simulink model "Verifikation_Dyn_R2019b"  (R2023a)
settings: Solver=ode5  StartTime=0.0  StopTime=10.0  FixedStep=Ta  RelTol=1e-3
values from neighbouring files (symbols this model uses):
  params_CRS = [g m2 m3 s2 s3 l2 l3 B_S1 A_S2 B_S2 C_S2 A_S3 B_S3 C_S3 i_G1 i_G2 i_G3 B_M1 C_M2 C_M3]    [init_CRS255_ss.m]
  x1_ic = zeros(6,1)    [init_CRS255_ss.m]
settings Model: Creator=Hoebarth  LastModifiedBy=Flo
settings SolverCC: AlgebraicLoopSolver=TrustRegion
settings DataIOCC: LimitDataPoints=on  SaveFormat=Array  SignalLoggingSaveFormat=ModelDataLogs  ReturnWorkspaceOutputs=off  SignalLoggingName=sigsOut
settings OptimizationCC: BooleanDataType=off  OptimizeBlockIOStorage=off  BufferReuse=off  GlobalBufferReuse=off  ExpressionFolding=off  ExpressionDepthLimit=2147483647  LocalBlockOutputs=off  InitFltsAndDblsToZero=on  LifeSpan=inf  OptimizeDataStoreBuffers=off  BusAssignmentInplaceUpdate=off
settings DebuggingCC: SaveWithParameterizedLinksMsg=none  UnderspecifiedInitializationDetection=Classic  MergeDetectMultiDrivingBlocksExec=none  SignalResolutionControl=TryResolveAllWithWarning  MultiTaskDSMMsg=warning  MultiTaskCondExecSysMsg=none  FcnCallInpInsideContextMsg=warning  UnconnectedInputMsg=warning  UnconnectedOutputMsg=warning  UnconnectedLineMsg=warning  StateNameClashWarn=warning  SFUnexpectedBacktrackingDiag=warning  SFNoUnconditionalDefaultTransitionDiag=warning  SFExecutionAtInitializationDiag=none  ArithmeticOperatorsInVariantConditions=warning
settings HardwareCC: ProdBitPerPointer=32  ProdBitPerSizeT=32  ProdBitPerPtrDiffT=32  ProdLargestAtomicFloat=None  ProdIntDivRoundTo=Undefined  ProdEndianess=Unspecified  ProdWordSize=32  ProdHWDeviceType=32-bit Generic  TargetUnknown=on
settings ModelReferenceCC: EnableRefExpFcnMdlSchedulingChecks=on  PropagateSignalLabelsOutOfModel=off
settings SFSimCC: SimUseLocalCustomCode=off  CustomCodeUndefinedFunction=UseInterfaceOnly
settings RTWCC: MakeCommand=make_wc  GenerateMakefile=off  TemplateMakefile=nt_msvc.tmf  RTWUseLocalCustomCode=off
settings CodeAppCC: StateflowObjectComments=on
settings GRTTargetCC: TargetFcnLib=ansi_tfl_tmw.mat  TargetLangStandard=C89/C90 (ANSI)  ModelReferenceCompliant=off  CompOptLevelCompliant=off  CombineOutputUpdateFcns=off  MatFileLogging=off  GRTInterface=on  UseToolchainInfoCompliant=off
settings ConfigComp: CovMetricSettings=dw  CovSaveCumulativeToWorkspaceVar=on  CovSaveSingleToWorkspaceVar=on  CovExternalEMLEnable=off

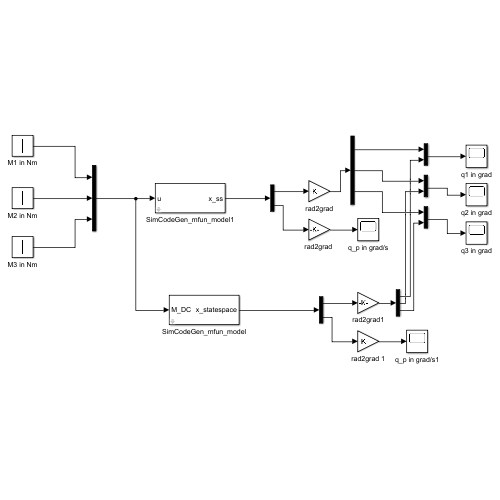
[thumbnail: Simulink's stored preview of the top-level diagram]
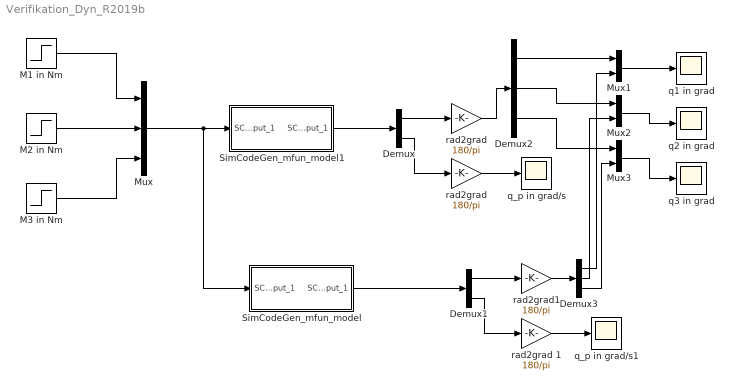
== system Verifikation_Dyn_R2019b ==
  Demux : Demux  Outputs=[3,3]
  Demux1 : Demux  Outputs=[3,3]
  Demux2 : Demux  Outputs=3
  Demux3 : Demux  Outputs=3
  M1 in Nm : Step  Before=0.001  After=0  SampleTime=0
  M2 in Nm : Step  Time=2  Before=0.001  After=0  SampleTime=0
  M3 in Nm : Step  Time=3  Before=0.001  After=0  SampleTime=0
  Mux : Mux  Inputs=3
  Mux1 : Mux  Inputs=2
  Mux2 : Mux  Inputs=2
  Mux3 : Mux  Inputs=2
  SimCodeGen_mfun_model : Subsystem  mask{SC_param_0=params_CRS, SC_x1_ic=x1_ic}
      mask prompts: SC_param_0 "params_CRS"
      mask Display:
      | port_label('input', 1, 'M_DC');
      | port_label('output', 1, 'x_statespace');
  SimCodeGen_mfun_model1 : Subsystem  mask{SC_param_0=params_CRS, SC_x1_ic=x1_ic}
      mask prompts: SC_param_0 "params_CRS"
      mask Display:
      | port_label('input', 1, 'u');
      | port_label('output', 1, 'x_ss');
  q1 in grad : Scope
  q2 in grad : Scope
  q3 in grad : Scope
  q_p in grad/s : Scope
  q_p in grad/s1 : Scope
  rad2grad : Gain  Gain=180/pi
  "rad2grad " : Gain  Gain=180/pi
  rad2grad 1 : Gain  Gain=180/pi
  rad2grad1 : Gain  Gain=180/pi
  wires:
  M1 in Nm/1 -> Mux/1
  M2 in Nm/1 -> Mux/2
  M3 in Nm/1 -> Mux/3
  Mux/1 -> SimCodeGen_mfun_model1/1(SC_input_1), SimCodeGen_mfun_model/1(SC_input_1)
  SimCodeGen_mfun_model1/1(SC_output_1) -> Demux/1
  Demux/1 -> rad2grad/1
  Demux/2 -> "rad2grad "/1
  "rad2grad "/1 -> q_p in grad/s/1
  rad2grad 1/1 -> q_p in grad/s1/1
  Demux1/2 -> rad2grad 1/1
  Demux1/1 -> rad2grad1/1
  SimCodeGen_mfun_model/1(SC_output_1) -> Demux1/1
  rad2grad/1 -> Demux2/1
  Demux2/1 -> Mux1/1
  Demux3/1 -> Mux1/2
  rad2grad1/1 -> Demux3/1
  Mux1/1 -> q1 in grad/1
  Demux2/2 -> Mux2/1
  Demux2/3 -> Mux3/1
  Demux3/2 -> Mux2/2
  Demux3/3 -> Mux3/2
  Mux2/1 -> q2 in grad/1
  Mux3/1 -> q3 in grad/1

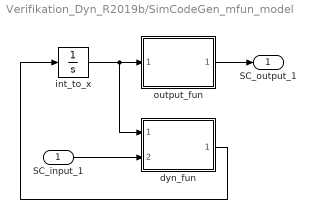
== system Verifikation_Dyn_R2019b/SimCodeGen_mfun_model ==
  SC_input_1 : Inport
  dyn_fun : MATLAB Function  TreatAsAtomicUnit=on
  int_to_x : Integrator  InitialCondition=[SC_x1_ic]
  output_fun : MATLAB Function  TreatAsAtomicUnit=on
  SC_output_1 : Outport
  wires:
  dyn_fun/1(SC_state_dot) -> int_to_x/1
  output_fun/1(SC_output_0) -> SC_output_1/1
  SC_input_1/1 -> dyn_fun/2(SC_input_0)
  int_to_x/1 -> output_fun/1(SC_state), dyn_fun/1(SC_state)

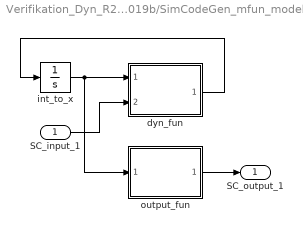
== system Verifikation_Dyn_R2019b/SimCodeGen_mfun_model1 ==
  SC_input_1 : Inport
  dyn_fun : MATLAB Function  TreatAsAtomicUnit=on
  int_to_x : Integrator  InitialCondition=[SC_x1_ic]
  output_fun : MATLAB Function  TreatAsAtomicUnit=on
  SC_output_1 : Outport
  wires:
  output_fun/1(SC_output_0) -> SC_output_1/1
  int_to_x/1 -> output_fun/1(SC_state), dyn_fun/1(SC_state)
  SC_input_1/1 -> dyn_fun/2(SC_input_0)
  dyn_fun/1(SC_state_dot) -> int_to_x/1

== matlab function Verifikation_Dyn_R2019b/SimCodeGen_mfun_model/dyn_fun ==
  data: SC_state input size=[6]; SC_state_dot output size=[6]; SC_input_0 input size=[3]; SC_param_0 parameter
function SC_state_dot  = dyn_fun(SC_state, SC_input_0, SC_param_0)
    SC_state_dot = zeros(6, 1);
    SC_state_x_0 = SC_state(1:6);
    SC_eval = zeros(6,1);
    SC_eval(1) = SC_state_x_0(4);
    SC_eval(2) = SC_state_x_0(5);
    SC_eval(3) = SC_state_x_0(6);
    t1 = SC_state_x_0(2);
    t2 = cos(t1);
    t3 = t2 ^ 2;
    t4 = SC_param_0(6);
    t5 = t4 ^ 2;
    t7 = SC_param_0(3);
    t9 = SC_param_0(2);
    t11 = SC_param_0(4);
    t12 = t11 ^ 2;
    t14 = sin(t1);
    t15 = SC_state_x_0(3);
    t16 = cos(t15);
    t19 = SC_param_0(5);
    t23 = t16 ^ 2;
    t25 = t19 ^ 2;
    t27 = SC_param_0(9);
    t29 = SC_param_0(12);
    t31 = SC_param_0(15);
    t32 = t31 ^ 2;
    t35 = SC_param_0(10);
    t37 = SC_param_0(13);
    t39 = t7 * t5;
    t40 = t9 * t12;
    t18 = t9 * t12;
    t21 = t25 * t7;
    t24 = t7 * t5;
    t42 = 0.2e1 * t14 * t16 * t19 * t4 * t7 - t18 * t3 + t21 * t23 - t23 * t29 + t23 * t37 - t24 * t3 + t27 * t3 - t3 * t35 + t32 * SC_param_0(18) + t29 + t35 + t39 + t40 + SC_param_0(8);
    t43 = SC_eval(2);
    t46 = t43 * t2;
    t50 = t27 * t43;
    t44 = SC_eval(1);
    t51 = t14 * t44;
    t53 = t43 * t35;
    t55 = SC_param_0(11);
    t56 = t55 * t43;
    t60 = t2 * t44;
    t68 = t14 * t4 + t16 * t19;
    t71 = sin(t15);
    t76 = t16 * t44;
    t78 = t1 + t15;
    t79 = cos(t78);
    t80 = t4 * t79;
    t81 = t80 * t43;
    t83 = t71 * t44;
    t84 = sin(t78);
    t85 = t4 * t84;
    t86 = t85 * t43;
    t48 = SC_eval(3);
    t88 = t19 * t48 - t86;
    t93 = t29 * t48;
    t95 = t48 * t37;
    t97 = SC_param_0(14);
    t98 = t97 * t48;
    SC_eval(4) = 0.1e1 / t42 * (-0.2e1 * t14 * t18 * t46 * t44 + (t50 * t51 - t51 * t53 + t51 * t56) * t2 + (t50 * t60 - t53 * t60 - t56 * t60) * t14 - t68 * (t7 * t44 * (-t19 * t48 * t71 + t4 * t46) + t81 * t7 * t76 - t88 * t7 * t83) + (-t76 * t93 + t76 * t95 - t76 * t98) * t71 + (-t83 * t93 + t83 * t95 + t83 * t98) * t16 + SC_input_0(1) * t31);
    t110 = t25 * t7;
    t111 = SC_param_0(17);
    t112 = t111 ^ 2;
    t113 = SC_param_0(20);
    t114 = t113 * t112;
    t116 = t84 ^ 2;
    t118 = t7 ^ 2;
    t121 = SC_param_0(19);
    t123 = SC_param_0(16);
    t124 = t123 ^ 2;
    t127 = t121 * t124;
    t125 = t25 * t118;
    t147 = t112 * t113 * t121 * t124 + t12 * t25 * t7 * t9 + t112 * t113 * t55 - t116 * t125 * t5 + t121 * t124 * t97 + t110 * t127 + t114 * t39 + t114 * t40 + t125 * t5 + t18 * t97 + t21 * t55 + t24 * t97 + t55 * t97;
    t148 = 0.1e1 / t147;
    t150 = t44 ^ 2;
    t151 = t150 * t2;
    t152 = t14 * t9;
    t155 = SC_param_0(1);
    t165 = t7 * (t43 + t48);
    t167 = t48 * t7;
    t169 = t150 * t16;
    t170 = t68 * t7;
    t178 = t150 * t71;
    t182 = t155 * t16 * t7 - t165 * t81 + t167 * t81 + t170 * t178;
    t186 = (t11 * t151 * t152 + t152 * t155) * t11 - t2 * t27 * t150 * t14 + t14 * t35 * t151 - (t155 * t7 * t71 - t165 * t86 - t167 * t88 - t169 * t170) * t80 + t182 * t85 + SC_input_0(2) * t123;
    t188 = t7 * t85;
    t189 = t148 * t19;
    t197 = -t16 * t178 * t37 + t169 * t29 * t71 + t111 * SC_input_0(3) - t182 * t19;
    SC_eval(5) = t186 * t148 * (t110 + t114 + t97) + t197 * t189 * t188;
    SC_eval(6) = t186 * t189 * t188 + t197 * t148 * (t40 + t39 + t127 + t55);
    SC_state_dot(1:6) = SC_eval(1:6);
end

== matlab function Verifikation_Dyn_R2019b/SimCodeGen_mfun_model1/dyn_fun ==
  data: SC_state input size=[6]; SC_state_dot output size=[6]; SC_input_0 input size=[3]; SC_param_0 parameter
function SC_state_dot  = dyn_fun(SC_state, SC_input_0, SC_param_0)
    SC_state_dot = zeros(6, 1);
    SC_state_x_0 = SC_state(1:6);
    SC_eval = zeros(6,1);
    SC_eval(1) = SC_state_x_0(4);
    SC_eval(2) = SC_state_x_0(5);
    SC_eval(3) = SC_state_x_0(6);
    t1 = SC_state_x_0(3);
    t2 = cos(t1);
    t3 = t2 ^ 2;
    t4 = SC_param_0(3);
    t6 = SC_param_0(5);
    t7 = t6 ^ 2;
    t9 = SC_param_0(6);
    t10 = t9 * t4;
    t11 = t2 * t6;
    t12 = SC_state_x_0(2);
    t13 = sin(t12);
    t17 = t13 ^ 2;
    t18 = t9 ^ 2;
    t21 = SC_param_0(2);
    t23 = SC_param_0(4);
    t24 = t23 ^ 2;
    t26 = SC_param_0(9);
    t27 = cos(t12);
    t28 = t27 ^ 2;
    t30 = SC_param_0(12);
    t31 = sin(t1);
    t32 = t31 ^ 2;
    t34 = SC_param_0(15);
    t35 = t34 ^ 2;
    t38 = SC_param_0(10);
    t40 = SC_param_0(13);
    t48 = t24 * t21;
    t49 = t18 * t4;
    t50 = t48 + t49 - t26 + t38;
    t56 = t4 * t6;
    t58 = t7 * t4;
    t59 = t58 - t30 + t40;
    t14 = SC_eval(1);
    t15 = SC_eval(2);
    t41 = SC_eval(3);
    t53 = t18 * t4;
    t55 = t24 * t21;
    t60 = t7 * t4;
    SC_eval(4) = 0.1e1 / (0.2e1 * t10 * t11 * t13 + t17 * t38 + t17 * t53 + t17 * t55 + t26 * t28 + t3 * t40 + t3 * t60 + t30 * t32 + t35 * SC_param_0(18) + SC_param_0(8)) * (t34 * SC_input_0(1) - 0.2e1 * ((t11 * t10 + t13 * t50) * t15 * t27 - t41 * (t13 * t56 * t9 + t2 * t59) * t31) * t14);
    t68 = SC_param_0(17);
    t69 = t68 ^ 2;
    t70 = SC_param_0(20);
    t71 = t70 * t69;
    t72 = SC_param_0(14);
    t74 = t1 + t12;
    t75 = sin(t74);
    t76 = t75 ^ 2;
    t78 = t4 ^ 2;
    t81 = SC_param_0(19);
    t83 = SC_param_0(16);
    t84 = t83 ^ 2;
    t87 = t81 * t84;
    t98 = SC_param_0(11);
    t80 = t7 * t78;
    t108 = t21 * t24 * t4 * t7 + t69 * t70 * t81 * t84 - t18 * t76 * t80 + t69 * t70 * t98 + t72 * t81 * t84 + t18 * t80 + t48 * t71 + t49 * t71 + t53 * t72 + t55 * t72 + t58 * t87 + t60 * t98 + t72 * t98;
    t109 = 0.1e1 / t108;
    t113 = t14 ^ 2;
    t116 = cos(-t1 + t12);
    t119 = t116 * t113 * t9 * t56 / 0.2e1;
    t122 = sin(0.2e1 * t12);
    t125 = t41 ^ 2;
    t129 = cos(t74);
    t133 = SC_param_0(1);
    t138 = t83 * SC_input_0(2) + t119 + t122 * t50 * t113 / 0.2e1 + t129 * (t113 + 0.2e1 * t125) * t6 * t10 / 0.2e1 + t13 * (t21 * t23 + t10) * t133;
    t140 = t75 * t56;
    t141 = t109 * t9;
    t146 = sin(0.2e1 * t1);
    t149 = t15 ^ 2;
    t158 = t68 * SC_input_0(3) - t119 - t146 * t59 * t113 / 0.2e1 - t6 * t4 * (-t129 * t9 * (t149 + t113 / 0.2e1) + t133 * t2);
    SC_eval(5) = t138 * t109 * (t58 + t71 + t72) + t158 * t141 * t140;
    SC_eval(6) = t138 * t141 * t140 + t158 * t109 * (t48 + t49 + t87 + t98);
    SC_state_dot(1:6) = SC_eval(1:6);
end

== matlab function Verifikation_Dyn_R2019b/SimCodeGen_mfun_model1/output_fun ==
  data: SC_state input size=[6]; SC_output_0 output size=[6]; SC_param_0 parameter size=[20]
function SC_output_0  = y_fun(SC_state, SC_param_0)
    SC_output_0 = zeros(6,1);
    SC_state_x_0 = SC_state(1:6);
    SC_output_0(1) = SC_state_x_0(1);
    SC_output_0(2) = SC_state_x_0(2);
    SC_output_0(3) = SC_state_x_0(3);
    SC_output_0(4) = SC_state_x_0(4);
    SC_output_0(5) = SC_state_x_0(5);
    SC_output_0(6) = SC_state_x_0(6);
end

== matlab function Verifikation_Dyn_R2019b/SimCodeGen_mfun_model/output_fun ==
  data: SC_state input size=[6]; SC_output_0 output size=[6]; SC_param_0 parameter size=[20]
function SC_output_0  = y_fun(SC_state, SC_param_0)
    SC_output_0 = zeros(6,1);
    SC_state_x_0 = SC_state(1:6);
    SC_output_0(1) = SC_state_x_0(1);
    SC_output_0(2) = SC_state_x_0(2);
    SC_output_0(3) = SC_state_x_0(3);
    SC_output_0(4) = SC_state_x_0(4);
    SC_output_0(5) = SC_state_x_0(5);
    SC_output_0(6) = SC_state_x_0(6);
end
